simulink model "passive"  (R2020a)
settings: Solver=VariableStepAuto  StartTime=0.0  StopTime=10.0  RelTol=1e-3
undefined symbols (not defined in the file): A, C, E, H, params
libraries: simulink x1
settings Model: Creator=lwb  LastModifiedBy=lwb
settings DebuggingCC: UnconnectedInputMsg=none  UnconnectedOutputMsg=none  UnconnectedLineMsg=none
settings ModelReferenceCC: EnableRefExpFcnMdlSchedulingChecks=off
settings RTWCC: Description=Generic Real-Time Target

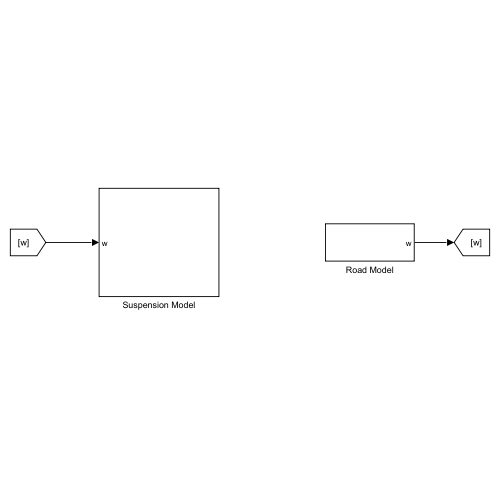
[thumbnail: Simulink's stored preview of the top-level diagram]
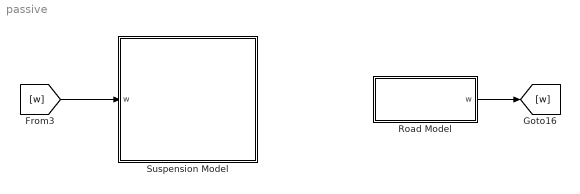
== system passive ==
  Road Model : Subsystem
  Suspension Model : Subsystem
  wires:
  Road Model/1(w) -> [w]
  [w] -> Suspension Model/1(w)

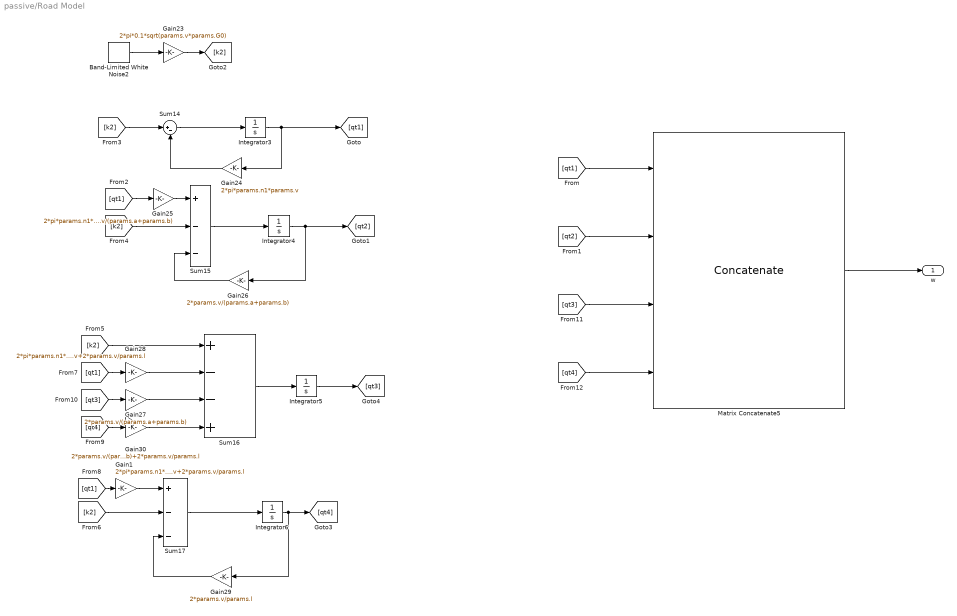
== system passive/Road Model ==
  Band-Limited White Noise2 : simulink/Sources/Band-Limited White Noise  Cov=[0.5]  Ts=1/10/params.v  seed=[23341]
  Gain1 : Gain  Gain=2*pi*params.n1*params.v+2*params.v/params.l
  Gain23 : Gain  Gain=2*pi*0.1*sqrt(params.v*params.G0)
  Gain24 : Gain  Gain=2*pi*params.n1*params.v
  Gain25 : Gain  Gain=2*pi*params.n1*params.v+2*params.v/(params.a+params.b)
  Gain26 : Gain  Gain=2*params.v/(params.a+params.b)
  Gain27 : Gain  Gain=2*params.v/(params.a+params.b)
  Gain28 : Gain  Gain=2*pi*params.n1*params.v+2*params.v/params.l
  Gain29 : Gain  Gain=2*params.v/params.l
  Gain30 : Gain  Gain=2*params.v/(params.a+params.b)+2*params.v/params.l
  Integrator{3..6} (4 alike) : Integrator
  Matrix Concatenate5 : Concatenate  NumInputs=4  Mode=Multidimensional array
  Sum14 : Sum  Inputs=|+-
  Sum15 : Sum  Inputs=+--
  Sum16 : Sum  Inputs=+--+
  Sum17 : Sum  Inputs=+--
  w : Outport
  wires:
  Gain25/1 -> Sum15/1
  Gain27/1 -> Sum16/3
  Gain26/1 -> Sum15/3
  Gain24/1 -> Sum14/2
  Integrator5/1 -> [qt3]
  Integrator3/1 -> Gain24/1, [qt1]
  Matrix Concatenate5/1 -> w/1
  Sum14/1 -> Integrator3/1
  Integrator4/1 -> Gain26/1, [qt2]
  Integrator6/1 -> Gain29/1, [qt4]
  Gain28/1 -> Sum16/2
  Gain29/1 -> Sum17/3
  Sum16/1 -> Integrator5/1
  Sum15/1 -> Integrator4/1
  Gain30/1 -> Sum16/4
  Sum17/1 -> Integrator6/1
  [k2] -> Sum14/1
  Band-Limited White Noise2/1 -> Gain23/1
  Gain23/1 -> [k2]
  [k2] -> Sum15/2
  [k2] -> Sum16/1
  [k2] -> Sum17/2
  [qt1] -> Gain25/1
  [qt1] -> Gain28/1
  [qt1] -> Gain1/1
  Gain1/1 -> Sum17/1
  [qt3] -> Gain27/1
  [qt4] -> Gain30/1
  [qt3] -> Matrix Concatenate5/3
  [qt4] -> Matrix Concatenate5/4
  [qt1] -> Matrix Concatenate5/1
  [qt2] -> Matrix Concatenate5/2

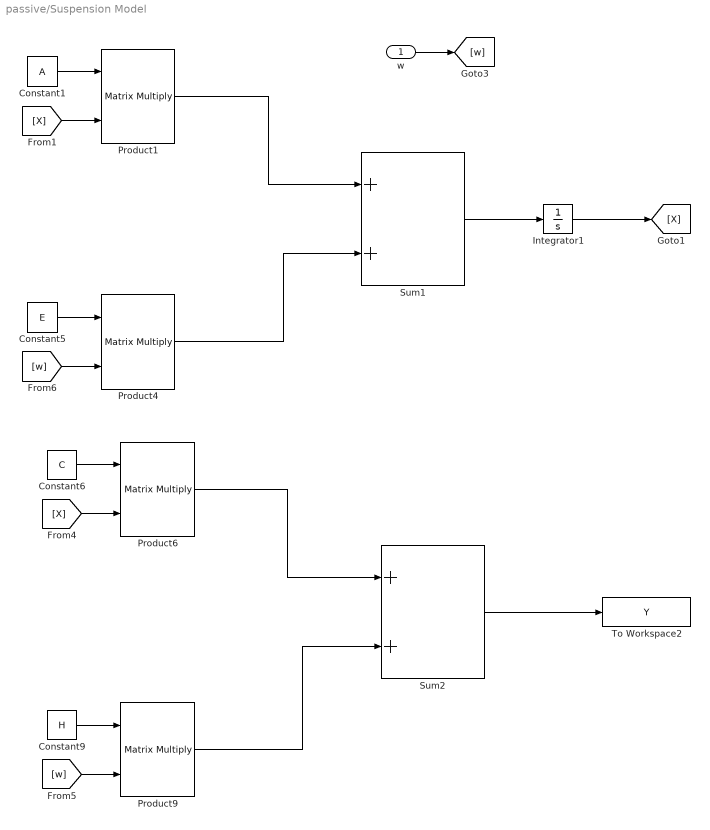
== system passive/Suspension Model ==
  w : Inport
  Constant1 : Constant  Value=A  VectorParams1D=off
  Constant5 : Constant  Value=E  VectorParams1D=off
  Constant6 : Constant  Value=C  VectorParams1D=off
  Constant9 : Constant  Value=H  VectorParams1D=off
  Integrator1 : Integrator
  Product{1,4,6,9} (4 alike) : Product  Multiplication=Matrix(*)
  Sum1 : Sum
  Sum2 : Sum
  To Workspace2 : ToWorkspace  VariableName=Y  SaveFormat=Timeseries  SampleTime=-1
  wires:
  Product4/1 -> Sum1/2
  Product1/1 -> Sum1/1
  Constant1/1 -> Product1/1
  Product6/1 -> Sum2/1
  Sum1/1 -> Integrator1/1
  Product9/1 -> Sum2/2
  [X] -> Product1/2
  [w] -> Product9/2
  Constant9/1 -> Product9/1
  Constant6/1 -> Product6/1
  Sum2/1 -> To Workspace2/1
  [X] -> Product6/2
  [w] -> Product4/2
  Constant5/1 -> Product4/1
  w/1 -> [w]
  Integrator1/1 -> [X]
